simulink model "pole_placement_2dof"  (R2023b)
settings: Solver=FixedStepAuto  StartTime=0.0  StopTime=Tend_slk*2  RelTol=1e-3
values from neighbouring files (symbols this model uses):
  Kv = K(:,5:6)    [main_pole_2dof.m]
  Kx = K(:,1:4)    [main_pole_2dof.m]
  param = [Ixx;Iyy;Izz;l;k;b;m]    [main_H2_2dof.m]    (also in main_inverse_2dof.m; main_pole_2dof.m)
  Ts_slk = 0.01    [main_H2_2dof.m]    (also in main_inverse_2dof.m; main_pole_2dof.m)
  x0 = [1;1;0;0]*0.01    [main_H2_2dof.m]    (also in main_inverse_2dof.m = [0;0;0;0]; main_pole_2dof.m)
  x_des = [1;1;0;0]    [main_H2_2dof.m]    (also in main_pole_2dof.m)
settings Model: Creator=asus  LastModifiedBy=asus
settings OptimizationCC: ReuseModelBlockBuffer=off

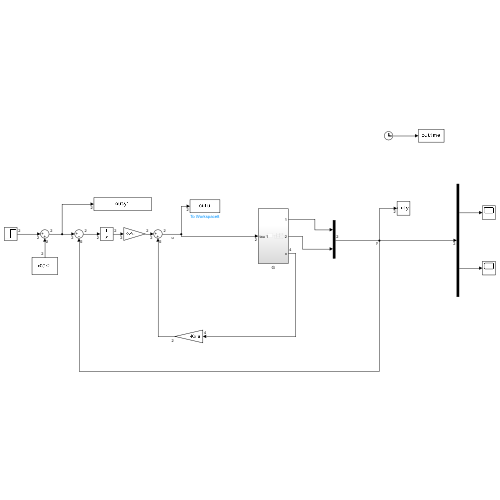
[thumbnail: Simulink's stored preview of the top-level diagram]
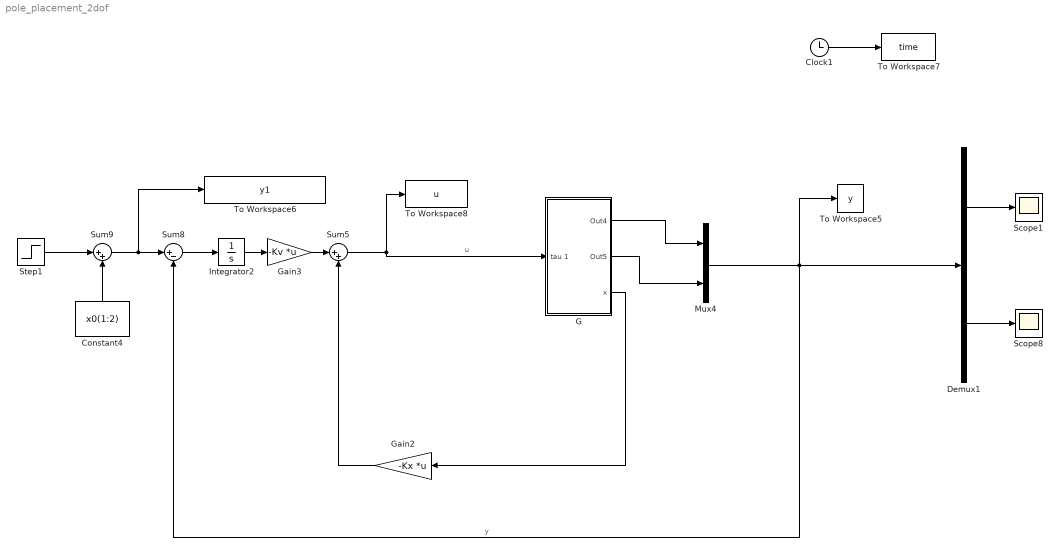
== system pole_placement_2dof ==
  Clock1 : Clock
  Constant4 : Constant  Value=x0(1:2)
  Demux1 : Demux  Outputs=2
  G : Subsystem
  Gain2 : Gain  Gain=-Kx  Multiplication=Matrix(K*u)
  Gain3 : Gain  Gain=-Kv  Multiplication=Matrix(K*u)
  Integrator2 : Integrator
  Mux4 : Mux  Inputs=2
  Scope1 : Scope
  Scope8 : Scope
  Step1 : Step  After=x_des(1:2)*30*pi/180  SampleTime=0
  Sum5 : Sum  Inputs=|++
  Sum8 : Sum  Inputs=|+-
  Sum9 : Sum  Inputs=|++
  To Workspace5 : ToWorkspace  VariableName=y  SampleTime=-1
      settings: Save2DSignal=2-D array (concatenate along first dimension)
  To Workspace6 : ToWorkspace  VariableName=y1  SampleTime=Ts_slk
  To Workspace7 : ToWorkspace  VariableName=time  SampleTime=Ts_slk
      settings: Save2DSignal=2-D array (concatenate along first dimension)
  To Workspace8 : ToWorkspace  VariableName=u  SampleTime=Ts_slk
  wires:
  Mux4/1 -> To Workspace5/1, Demux1/1, Sum8/2  "y"
  G/3(x) -> Gain2/1
  Sum8/1 -> Integrator2/1
  Gain2/1 -> Sum5/2
  Demux1/2 -> Scope8/1
  Gain3/1 -> Sum5/1
  Sum9/1 -> To Workspace6/1, Sum8/1
  Sum5/1 -> To Workspace8/1, G/1(tau 1)  "u"
  Constant4/1 -> Sum9/2
  Clock1/1 -> To Workspace7/1
  Integrator2/1 -> Gain3/1
  Step1/1 -> Sum9/1
  Demux1/1 -> Scope1/1
  G/1(Out4) -> Mux4/1
  G/2(Out5) -> Mux4/2

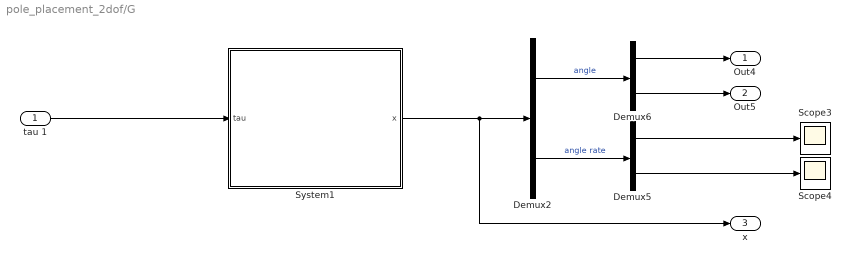
== system pole_placement_2dof/G ==
  tau 1 : Inport
  Demux2 : Demux  Outputs=2
  Demux5 : Demux  Outputs=2
  Demux6 : Demux  Outputs=2
  Scope3 : Scope
  Scope4 : Scope
  System1 : Subsystem
  Out4 : Outport
  Out5 : Outport  Port=2
  x : Outport  Port=3
  wires:
  Demux5/1 -> Scope3/1
  Demux6/1 -> Out4/1
  Demux6/2 -> Out5/1
  tau 1/1 -> System1/1("tau ")
  Demux5/2 -> Scope4/1
  System1/1(x) -> x/1, Demux2/1
  Demux2/2 -> Demux5/1  "angle rate"
  Demux2/1 -> Demux6/1  "angle"

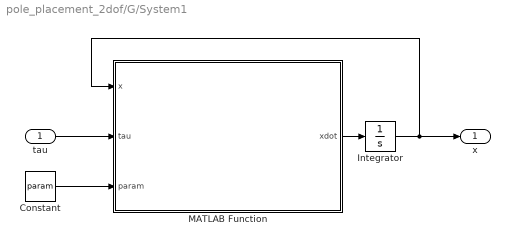
== system pole_placement_2dof/G/System1 ==
  "tau " : Inport
  Constant : Constant  Value=param
  Integrator : Integrator  InitialCondition=x0
  MATLAB Function : MATLAB Function  TreatAsAtomicUnit=on
  x : Outport
  wires:
  Integrator/1 -> MATLAB Function/1(x), x/1
  MATLAB Function/1(xdot) -> Integrator/1
  "tau "/1 -> MATLAB Function/2(tau)
  Constant/1 -> MATLAB Function/3(param)

== matlab function pole_placement_2dof/G/System1/MATLAB Function ==
  data: x input; tau input; xdot output; param input
function xdot =quadcopter(x,tau,param)
% Inputs:
%           x       (model state)
%           tau     (torque)           
%           param   (model parameters)
%
% Outputs:  x_dot  (derivative of the state with respect to time)

% Parameters
g        =       9.81;           %  gravity acceleration (m/s^2)
Ixx      =       param(1,1);     %  moment of inertia 
Iyy      =       param(2,1);     %  moment of inertia
Izz      =       param(3,1);     %  moment of inertia 

% States
phi      =       x(1,1);     %  roll angle (rad)
theta    =       x(2,1);     %  pitch angle (rad)
phi_dot  =       x(3,1);     %  roll rate (rad/s)
theta_dot=       x(4,1);     %  pitch rate (rad/s)

cph         =       cos(phi);
cth         =       cos(theta);
sph         =       sin(phi);
sth         =       sin(theta);

% torques
tau_1    =       tau(1,1);   %  roll torque 
tau_2    =       tau(2,1);   %  pitch torque  

% Coriolis matrix
C11=  0;
C12= (Iyy)*(theta_dot*cph*sph);
C21= (Iyy)*(theta_dot*cph*sph);
C22= 0;

C  = [C11 C12;
      C21 C22];

% Inertia matrix
J11= Ixx;
J12= 0;
J21= 0;
J22= Iyy*cph^2;

J  = [J11 J12;
     J21 J22];

%% Model Equation 
invJ = [ J22/(J11*J22 - J12*J21), -J12/(J11*J22 - J12*J21);
        -J21/(J11*J22 - J12*J21),  J11/(J11*J22 - J12*J21)];

xdot        = zeros(4,1);
xdot(1:2,1) = x(3:4,1);
xdot(3:4,1) = invJ*(tau - C*x(3:4,1));
